simulink model "Voltage_Monitor_Latch_Model"  (R2025a)
settings: Solver=VariableStepAuto  StartTime=0.0  StopTime=10.0  RelTol=1e-3
libraries: simulink x1
settings Model: Creator=mahij  LastModifiedBy=mahij

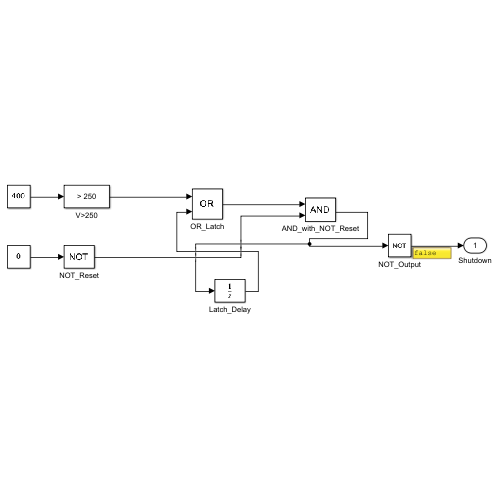
[thumbnail: Simulink's stored preview of the top-level diagram]
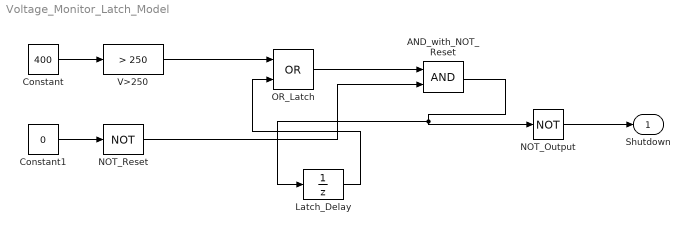
== system Voltage_Monitor_Latch_Model ==
  AND_with_NOT_Reset : Logic  AllPortsSameDT=off  OutDataTypeStr=boolean
  Constant : Constant  Value=400
  Constant1 : Constant  Value=0
  Latch_Delay : UnitDelay  SampleTime=-1  HasFrameUpgradeWarning=on
  NOT_Output : Logic  Operator=NOT  AllPortsSameDT=off  OutDataTypeStr=boolean
  NOT_Reset : Logic  Operator=NOT  AllPortsSameDT=off  OutDataTypeStr=boolean
  OR_Latch : Logic  Operator=OR  AllPortsSameDT=off  OutDataTypeStr=boolean
  V>250 : simulink/Logic and Bit Operations/Compare To Constant  relop=>  const=250  OutDataTypeStr=boolean
  Shutdown : Outport
  wires:
  Constant/1 -> V>250/1
  Constant1/1 -> NOT_Reset/1
  V>250/1 -> OR_Latch/1
  Latch_Delay/1 -> OR_Latch/2
  OR_Latch/1 -> AND_with_NOT_Reset/1
  NOT_Reset/1 -> AND_with_NOT_Reset/2
  AND_with_NOT_Reset/1 -> Latch_Delay/1, NOT_Output/1
  NOT_Output/1 -> Shutdown/1
